simulink model "Robot"  (R2018a)
settings: Solver=VariableStepAuto  StartTime=0.0  StopTime=inf  FixedStep=1e-4  RelTol=1e-3  EnableMultiTasking=on
values from neighbouring files (symbols this model uses):
  CM730_acc_center = (4 * 9.80665)    (= 39.2266)    [CM730.m]
  CM730_acc_gain = 512 / CM730_acc_center    (= 13.0523675261)    [CM730.m]
  CM730_gyro_center = (1600 / 360 * 2 * pi)    (= 27.9252680319)    [CM730.m]
  CM730_gyro_gain = 512 / CM730_gyro_center    (= 18.3346494442)    [CM730.m]
  CM730_sample_time = 1e-3    (= 0.001)    [CM730.m]
  FSR_max = 254    [FSR.m]
  FSR_no_load = 255    [FSR.m]
  FSR_sample_time = 0.001    [FSR.m]
  FSR_scale = 1000    [FSR.m]
  g = 0    [Euler.m]
  MX106_Te = 1/1000    (= 0.001)    [MX106_init.m]
  MX28_inertia = 9e-8 * MX28_reduction^2    (= 0.0033385284)    [MX28_init.m]
  MX28_Te = 1/1000    (= 0.001)    [MX28_init.m]
  posZero_ID1 = posZero(1)    [Robot_init.m]
  posZero_ID10 = posZero(14)    [Robot_init.m]
  posZero_ID11 = posZero(9)    [Robot_init.m]
  posZero_ID12 = posZero(15)    [Robot_init.m]
  posZero_ID13 = posZero(10)    [Robot_init.m]
  posZero_ID14 = posZero(16)    [Robot_init.m]
  posZero_ID15 = posZero(11)    [Robot_init.m]
  posZero_ID16 = posZero(17)    [Robot_init.m]
  posZero_ID17 = posZero(12)    [Robot_init.m]
  posZero_ID18 = posZero(18)    [Robot_init.m]
  posZero_ID19 = posZero(19)    [Robot_init.m]
  posZero_ID2 = posZero(4)    [Robot_init.m]
  posZero_ID20 = posZero(20)    [Robot_init.m]
  posZero_ID3 = posZero(2)    [Robot_init.m]
  posZero_ID4 = posZero(5)    [Robot_init.m]
  posZero_ID5 = posZero(3)    [Robot_init.m]
  posZero_ID6 = posZero(6)    [Robot_init.m]
  posZero_ID7 = posZero(7)    [Robot_init.m]
  posZero_ID8 = posZero(13)    [Robot_init.m]
  posZero_ID9 = posZero(8)    [Robot_init.m]
  robot_chest_mass = 2385.0    (= 2385)    [Robot_init.m]
  robot_floor_friction_coeff = 0.6    [Robot_init.m]
  robot_floor_position_gain = -1e5    (= -100000)    [Robot_init.m]
  robot_floor_speed_gain = -1e3    (= -1000)    [Robot_init.m]
  robot_gravity = [0 0 0]    [Robot_init.m]
  robot_head_mass = 177.69    [Robot_init.m]
  robot_hip1_mass = 49.00    (= 49)    [Robot_init.m]
  robot_left_ankle_mass = 360.00    (= 360)    [Robot_init.m]
  robot_left_foot_mass = 267.00    (= 267)    [Robot_init.m]
  robot_left_forearm_mass = 248.00    (= 248)    [Robot_init.m]
  robot_left_hip2_mass = 358.00    (= 358)    [Robot_init.m]
  robot_left_lower_leg_mass = 129.00    (= 129)    [Robot_init.m]
  robot_left_shoulder_mass = 39.00    (= 39)    [Robot_init.m]
  robot_left_thigh_mass = 1263.00    (= 1263)    [Robot_init.m]
  robot_left_upper_arm_mass = 247.00    (= 247)    [Robot_init.m]
  robot_neck_mass = 90    [Robot_init.m]
  robot_right_ankle_mass = 360.00    (= 360)    [Robot_init.m]
  robot_right_foot_mass = 267.00    (= 267)    [Robot_init.m]
  robot_right_forearm_mass = 248.00    (= 248)    [Robot_init.m]
  robot_right_hip2_mass = 358.00    (= 358)    [Robot_init.m]
  robot_right_lower_leg_mass = 129.00    (= 129)    [Robot_init.m]
  robot_right_shoulder_mass = 39.00    (= 39)    [Robot_init.m]
  robot_right_thigh_mass = 263.00    (= 263)    [Robot_init.m]
  robot_right_upper_arm_mass = 247.00    (= 247)    [Robot_init.m]
  X = get(hObject,'Value')    [gui_kine.m]
  Y = get(hObject,'Value')    [gui_kine.m]
  Z = get(hObject,'Value')    [gui_kine.m]
libraries: sm_lib x167, fl_lib x128, nesl_utility x77, dspindex x1
(part 4 of 7)

== system Robot/Robot simulation/Left Leg/Left Foot ==
  Left Foot Axis to Back Left : sm_lib/Frames and Transforms/Rigid Transform  TranslationMethod=Cartesian  TranslationStandardOffset=0  TranslationLengthUnit=mm  TranslationStandardAxis=+Z  TranslationCartesianOffset=robot_left_foot_to_back_left_floor_tra  TranslationROffset=0  TranslationROffsetUnits=m  TranslationZOffset=0  TranslationZOffsetUnits=m  TranslationThetaOffset=0  TranslationThetaOffsetUnits=deg  RotationMethod=RotationMatrix  RotationAngleUnits=deg  RotationStandardAxis=+Z  RotationAngle=0.0  RotationArbitraryAxis=[0 0 1]  FollAlignAxisA=+X  BaseAlignAxisA=-X  FollAlignAxisB=+Z  BaseAlignAxisB=-Y  RotationSequenceAxes=FollowerAxes  RotationSequence=XYX  RotationSequenceAngles=[0 0 0]  RotationSequenceAnglesUnits=deg  RotationMatrix=robot_left_foot_to_floor_rot
  Left Foot Axis to Back Right : sm_lib/Frames and Transforms/Rigid Transform  TranslationMethod=Cartesian  TranslationStandardOffset=0  TranslationLengthUnit=mm  TranslationStandardAxis=+Z  TranslationCartesianOffset=robot_left_foot_to_back_right_floor_tra  TranslationROffset=0  TranslationROffsetUnits=m  TranslationZOffset=0  TranslationZOffsetUnits=m  TranslationThetaOffset=0  TranslationThetaOffsetUnits=deg  RotationMethod=RotationMatrix  RotationAngleUnits=deg  RotationStandardAxis=+Z  RotationAngle=0.0  RotationArbitraryAxis=[0 0 1]  FollAlignAxisA=+X  BaseAlignAxisA=-X  FollAlignAxisB=+Z  BaseAlignAxisB=-Y  RotationSequenceAxes=FollowerAxes  RotationSequence=XYX  RotationSequenceAngles=[0 0 0]  RotationSequenceAnglesUnits=deg  RotationMatrix=robot_left_foot_to_floor_rot
  Left Foot Axis to Front Left : sm_lib/Frames and Transforms/Rigid Transform  TranslationMethod=Cartesian  TranslationStandardOffset=0  TranslationLengthUnit=mm  TranslationStandardAxis=+Z  TranslationCartesianOffset=robot_left_foot_to_front_left_floor_tra  TranslationROffset=0  TranslationROffsetUnits=m  TranslationZOffset=0  TranslationZOffsetUnits=m  TranslationThetaOffset=0  TranslationThetaOffsetUnits=deg  RotationMethod=RotationMatrix  RotationAngleUnits=deg  RotationStandardAxis=+Z  RotationAngle=0.0  RotationArbitraryAxis=[0 0 1]  FollAlignAxisA=+X  BaseAlignAxisA=-X  FollAlignAxisB=+Z  BaseAlignAxisB=-Y  RotationSequenceAxes=FollowerAxes  RotationSequence=XYX  RotationSequenceAngles=[0 0 0]  RotationSequenceAnglesUnits=deg  RotationMatrix=robot_left_foot_to_floor_rot
  Left Foot Axis to Front Right : sm_lib/Frames and Transforms/Rigid Transform  TranslationMethod=Cartesian  TranslationStandardOffset=0  TranslationLengthUnit=mm  TranslationStandardAxis=+Z  TranslationCartesianOffset=robot_left_foot_to_front_right_floor_tra  TranslationROffset=0  TranslationROffsetUnits=m  TranslationZOffset=0  TranslationZOffsetUnits=m  TranslationThetaOffset=0  TranslationThetaOffsetUnits=deg  RotationMethod=RotationMatrix  RotationAngleUnits=deg  RotationStandardAxis=+Z  RotationAngle=0.0  RotationArbitraryAxis=[0 0 1]  FollAlignAxisA=+X  BaseAlignAxisA=-X  FollAlignAxisB=+Z  BaseAlignAxisB=-Y  RotationSequenceAxes=FollowerAxes  RotationSequence=XYX  RotationSequenceAngles=[0 0 0]  RotationSequenceAnglesUnits=deg  RotationMatrix=robot_left_foot_to_floor_rot
  Left Foot Endefector : sm_lib/Frames and Transforms/Rigid Transform  TranslationMethod=Cartesian  TranslationStandardOffset=0  TranslationLengthUnit=mm  TranslationStandardAxis=+Z  TranslationCartesianOffset=robot_left_foot_Endefector_tra  TranslationROffset=0  TranslationROffsetUnits=m  TranslationZOffset=0  TranslationZOffsetUnits=m  TranslationThetaOffset=0  TranslationThetaOffsetUnits=deg  RotationMethod=RotationMatrix  RotationAngleUnits=deg  RotationStandardAxis=+Z  RotationAngle=0.0  RotationArbitraryAxis=[0 0 1]  FollAlignAxisA=+X  BaseAlignAxisA=-X  FollAlignAxisB=+Z  BaseAlignAxisB=-Y  RotationSequenceAxes=FollowerAxes  RotationSequence=XYX  RotationSequenceAngles=[0 0 0]  RotationSequenceAnglesUnits=deg  RotationMatrix=robot_left_foot_Endefector_rot
  Solid : sm_lib/Body Elements/Solid  InertiaType=Custom  Mass=robot_left_foot_mass  MassUnits=g  CenterOfMass=robot_left_foot_to_center_mass  CenterOfMassUnits=mm  MomentsOfInertia=robot_left_foot_moment_inertia  MomentsOfInertiaUnits=g*mm^2  ProductsOfInertia=robot_left_foot_product_inertia  ProductsOfInertiaUnits=g*mm^2  DensityBased=on  Density=1000  DensityUnits=kg/(m^3)  DoExposeReferenceFrame=on  SerializedFrames=<Frames/>  GraphicType=FromGeometry  MarkerShape=Sphere  MarkerSize=10  MarkerSizeUnits=m  GraphicVisPropType=SimpleVisualProperties  GraphicDiffuseColor=[0.5 0.5 0.5]  GraphicSpecularColor=[0.5 0.5 0.5 1.0]  GraphicAmbientColor=[0.15 0.15 0.15 1.0]  GraphicEmissiveColor=[0.0 0.0 0.0 1.0]  GraphicShininess=75  GraphicOpacity=1.0  GeometryShape=FromFile  RectangleSize=[1 1]  RectangleSizeUnits=m  BrickDimensions=[1 1 1]  BrickDimensionUnits=m  CylinderRadius=1  CylinderRadiusUnits=m  CylinderLength=1  CylinderLengthUnits=m  SphereRadius=1  SphereRadiusUnits=m  EllipsoidRadii=[1 1 1]  EllipsoidRadiiUnits=m  ExtrusionCrossSection=[1 1; -1 1; -1 -1; 1 -1]  ExtrusionCrossSectionUnits=m  ExtrusionLength=1  ExtrusionLengthUnits=m  PolygonNumSides=3  PolygonOuterRadius=1  PolygonOuterRadiusUnits=m  ExtGeomFileType=STL  ExtGeomFileName=\STL\Left_Foot.STL  ExtGeomFileUnits=mm  RevolutionCrossSection=[1 1; 1 -1; 2 -1; 2 1]  RevolutionCrossSectionUnits=m  RevolutionExtent=Full  RevolutionAngle=180  RevolutionAngleUnits=deg
  Foot : PMIOPort  Side=Left
  Front Left : PMIOPort  Port=2  Side=Right
  Front Right : PMIOPort  Port=3  Side=Right
  Back Right : PMIOPort  Port=4  Side=Right
  Back Left : PMIOPort  Port=5  Side=Right
  EndEfector : PMIOPort  Port=6  Side=Right
  connections:
  Foot/RConn1 -- Left Foot Axis to Back Right/LConn1 -- Left Foot Axis to Front Left/LConn1 -- Left Foot Endefector/LConn1 -- Left Foot Axis to Front Right/LConn1 -- Left Foot Axis to Back Left/LConn1 -- Solid/RConn1
  Front Left/RConn1 -- Left Foot Axis to Front Left/RConn1
  Front Right/RConn1 -- Left Foot Axis to Front Right/RConn1
  Back Right/RConn1 -- Left Foot Axis to Back Right/RConn1
  Back Left/RConn1 -- Left Foot Axis to Back Left/RConn1
  EndEfector/RConn1 -- Left Foot Endefector/RConn1

== system Robot/Robot simulation/Left Leg/Left Hip Pitch (12) ==
  Inertia : sm_lib/Body Elements/Inertia  InertiaType=Custom  Mass=1  MassUnits=g  CenterOfMass=[0 0 0]  CenterOfMassUnits=m  MomentsOfInertia=[0 0 MX28_inertia]  MomentsOfInertiaUnits=kg*m^2  ProductsOfInertia=[0 0 0]  ProductsOfInertiaUnits=kg*m^2  GraphicType=Marker  MarkerShape=Inertia  MarkerSize=20  GraphicVisPropType=SimpleVisualProperties  GraphicDiffuseColor=[0.5 0.5 0.5]  GraphicSpecularColor=[0.5 0.5 0.5 1.0]  GraphicAmbientColor=[0.15 0.15 0.15 1.0]  GraphicEmissiveColor=[0.0 0.0 0.0 1.0]  GraphicShininess=75  GraphicOpacity=1.0
  MX106 Command : DataStoreRead  DataStoreName=MX106_ID12  SampleTime=MX106_Te  DataStoreElements=MX106_ID12.CW_angle_limit#MX106_ID12.CCW_angle_limit#MX106_ID12.torque_enable#MX106_ID12.D_gain#MX106_ID12.I_gain#MX106_ID12.P_gain#MX106_ID12.goal_position#MX106_ID12.moving_speed#MX106_ID12.torque_limit
  MX106 State : DataStoreWrite  DataStoreName=MX106_ID12  DataStoreElements=MX106_ID12.present_position#MX106_ID12.present_speed#MX106_ID12.present_load#MX106_ID12.moving#MX106_ID12.pwm
  Model : ModelReference  ModelNameDialog=MX106.slx  SimulationMode=Normal  ModelReferenceVersion=1.67
  Position converter : nesl_utility/PS-Simulink Converter  PhysicalDomain=network_engine_domain  SubClassName=ps_output  LeftPortType=input  RightPortType=output  PseudoPeriodic=off  Frequencies=[]  Unit=rad  AffineConversion=off
  Revolute Joint : sm_lib/Joints/Revolute Joint  SenseConstraintForce=off  SenseConstraintForceX=off  SenseConstraintForceY=off  SenseConstraintForceZ=off  SenseConstraintTorque=off  SenseConstraintTorqueX=off  SenseConstraintTorqueY=off  SenseConstraintTorqueZ=off  SenseTotalForce=off  SenseTotalForceX=off  SenseTotalForceY=off  SenseTotalForceZ=off  SenseTotalTorque=off  SenseTotalTorqueX=off  SenseTotalTorqueY=off  SenseTotalTorqueZ=off  CompositeWrenchDir=FollowerOnBase  CompositeWrenchFrame=BaseFrame  EquilibriumPosition=0  EquilibriumPositionUnits=deg  SpringStiffness=0  SpringStiffnessUnits=N*m/deg  DampingCoefficient=MX28_lub_friction  DampingCoefficientUnits=N*m/(rad/s)  TorqueActuationMode=InputTorque  MotionActuationMode=ComputedMotion  SensePosition=on  SenseVelocity=on  SenseAcceleration=off  SenseTorqueForce=off  PositionTargetSpecify=on  PositionTargetPriority=High  PositionTargetValue=MX28_init_position  PositionTargetValueUnits=rad  VelocityTargetSpecify=on  VelocityTargetPriority=High  VelocityTargetValue=MX28_init_speed  VelocityTargetValueUnits=rad/s
  Speed converter : nesl_utility/PS-Simulink Converter  PhysicalDomain=network_engine_domain  SubClassName=ps_output  LeftPortType=input  RightPortType=output  PseudoPeriodic=off  Frequencies=[]  Unit=rad/s  AffineConversion=off
  Torque converter : nesl_utility/Simulink-PS Converter  PhysicalDomain=network_engine_domain  SubClassName=ps_input  LeftPortType=input  RightPortType=output  PseudoPeriodic=off  Frequencies=[]  NoiseDistribution=none  NoiseParameters=[]  Unit=N*m  AffineConversion=off  FilteringAndDerivatives=zero  SimscapeFilterOrder=1  InputFilterTimeConstant=0.001  UdotUserProvided=1
  Base : PMIOPort  Side=Left
  Axis : PMIOPort  Port=2  Side=Right
  wires:
  Model/4 -> MX106 State/3
  Model/2 -> MX106 State/1
  Model/5 -> MX106 State/4
  Model/3 -> MX106 State/2
  MX106 Command/3 -> Model/5
  MX106 Command/6 -> Model/8
  MX106 Command/4 -> Model/6
  MX106 Command/5 -> Model/7
  MX106 Command/7 -> Model/9
  MX106 Command/2 -> Model/4
  MX106 Command/1 -> Model/3
  Speed converter/1 -> Model/1
  Position converter/1 -> Model/2
  Model/6 -> MX106 State/5
  MX106 Command/8 -> Model/10
  MX106 Command/9 -> Model/11
  Model/1 -> Torque converter/1
  connections:
  Axis/RConn1 -- Revolute Joint/RConn1 -- Inertia/RConn1
  Revolute Joint/LConn1 -- Base/RConn1
  Revolute Joint/RConn3 -- Speed converter/LConn1
  Revolute Joint/RConn2 -- Position converter/LConn1
  Revolute Joint/LConn2 -- Torque converter/RConn1

== system Robot/Robot simulation/Left Leg/Left Hip Roll ==
  Left Hip Roll Base to Left Hip Pitch Base : sm_lib/Frames and Transforms/Rigid Transform  TranslationMethod=Cartesian  TranslationStandardOffset=0  TranslationLengthUnit=mm  TranslationStandardAxis=+Z  TranslationCartesianOffset=robot_left_hip2_to_left_thigh_tra  TranslationROffset=0  TranslationROffsetUnits=m  TranslationZOffset=0  TranslationZOffsetUnits=m  TranslationThetaOffset=0  TranslationThetaOffsetUnits=deg  RotationMethod=RotationMatrix  RotationAngleUnits=deg  RotationStandardAxis=+Z  RotationAngle=0  RotationArbitraryAxis=[0 0 1]  FollAlignAxisA=+Y  BaseAlignAxisA=+Y  FollAlignAxisB=+X  BaseAlignAxisB=+Z  RotationSequenceAxes=FollowerAxes  RotationSequence=XYX  RotationSequenceAngles=[0 0 0]  RotationSequenceAnglesUnits=deg  RotationMatrix=robot_left_hip2_to_left_thigh_rot
  Solid : sm_lib/Body Elements/Solid  InertiaType=Custom  Mass=robot_left_hip2_mass  MassUnits=g  CenterOfMass=robot_left_hip2_to_center_mass  CenterOfMassUnits=mm  MomentsOfInertia=robot_left_hip2_moment_inertia  MomentsOfInertiaUnits=g*mm^2  ProductsOfInertia=robot_left_hip2_product_inertia  ProductsOfInertiaUnits=g*mm^2  DensityBased=on  Density=1000  DensityUnits=kg/(m^3)  DoExposeReferenceFrame=on  SerializedFrames=<Frames/>  GraphicType=FromGeometry  MarkerShape=Sphere  MarkerSize=10  MarkerSizeUnits=m  GraphicVisPropType=SimpleVisualProperties  GraphicDiffuseColor=[0.5 0.5 0.5]  GraphicSpecularColor=[0.5 0.5 0.5 1.0]  GraphicAmbientColor=[0.15 0.15 0.15 1.0]  GraphicEmissiveColor=[0.0 0.0 0.0 1.0]  GraphicShininess=75  GraphicOpacity=1.0  GeometryShape=FromFile  RectangleSize=[1 1]  RectangleSizeUnits=m  BrickDimensions=[1 1 1]  BrickDimensionUnits=mm  CylinderRadius=1  CylinderRadiusUnits=m  CylinderLength=1  CylinderLengthUnits=m  SphereRadius=1  SphereRadiusUnits=m  EllipsoidRadii=[1 1 1]  EllipsoidRadiiUnits=m  ExtrusionCrossSection=[1 1; -1 1; -1 -1; 1 -1]  ExtrusionCrossSectionUnits=m  ExtrusionLength=1  ExtrusionLengthUnits=m  PolygonNumSides=3  PolygonOuterRadius=1  PolygonOuterRadiusUnits=m  ExtGeomFileType=STL  ExtGeomFileName=\STL\Left_Hip2.STL  ExtGeomFileUnits=mm  RevolutionCrossSection=[1 1; 1 -1; 2 -1; 2 1]  RevolutionCrossSectionUnits=m  RevolutionExtent=Full  RevolutionAngle=180  RevolutionAngleUnits=deg
  Left Hip Roll : PMIOPort  Side=Left
  Left Hip Pitch : PMIOPort  Port=2  Side=Right
  connections:
  Left Hip Roll Base to Left Hip Pitch Base/LConn1 -- Solid/RConn1 -- Left Hip Roll/RConn1
  Left Hip Roll Base to Left Hip Pitch Base/RConn1 -- Left Hip Pitch/RConn1

== system Robot/Robot simulation/Left Leg/Left Hip Roll (10) ==
  Inertia : sm_lib/Body Elements/Inertia  InertiaType=Custom  Mass=1  MassUnits=g  CenterOfMass=[0 0 0]  CenterOfMassUnits=m  MomentsOfInertia=[0 0 MX28_inertia]  MomentsOfInertiaUnits=kg*m^2  ProductsOfInertia=[0 0 0]  ProductsOfInertiaUnits=kg*m^2  GraphicType=Marker  MarkerShape=Inertia  MarkerSize=20  GraphicVisPropType=SimpleVisualProperties  GraphicDiffuseColor=[0.5 0.5 0.5]  GraphicSpecularColor=[0.5 0.5 0.5 1.0]  GraphicAmbientColor=[0.15 0.15 0.15 1.0]  GraphicEmissiveColor=[0.0 0.0 0.0 1.0]  GraphicShininess=75  GraphicOpacity=1.0
  MX106 Command : DataStoreRead  DataStoreName=MX106_ID10  SampleTime=MX106_Te  DataStoreElements=MX106_ID10.CW_angle_limit#MX106_ID10.CCW_angle_limit#MX106_ID10.torque_enable#MX106_ID10.D_gain#MX106_ID10.I_gain#MX106_ID10.P_gain#MX106_ID10.goal_position#MX106_ID10.moving_speed#MX106_ID10.torque_limit
  MX106 State : DataStoreWrite  DataStoreName=MX106_ID10  DataStoreElements=MX106_ID10.present_position#MX106_ID10.present_speed#MX106_ID10.present_load#MX106_ID10.moving#MX106_ID10.pwm
  Model : ModelReference  ModelNameDialog=MX106.slx  SimulationMode=Normal  ModelReferenceVersion=1.67
  Position converter : nesl_utility/PS-Simulink Converter  PhysicalDomain=network_engine_domain  SubClassName=ps_output  LeftPortType=input  RightPortType=output  PseudoPeriodic=off  Frequencies=[]  Unit=rad  AffineConversion=off
  Revolute Joint : sm_lib/Joints/Revolute Joint  SenseConstraintForce=off  SenseConstraintForceX=off  SenseConstraintForceY=off  SenseConstraintForceZ=off  SenseConstraintTorque=off  SenseConstraintTorqueX=off  SenseConstraintTorqueY=off  SenseConstraintTorqueZ=off  SenseTotalForce=off  SenseTotalForceX=off  SenseTotalForceY=off  SenseTotalForceZ=off  SenseTotalTorque=off  SenseTotalTorqueX=off  SenseTotalTorqueY=off  SenseTotalTorqueZ=off  CompositeWrenchDir=FollowerOnBase  CompositeWrenchFrame=BaseFrame  EquilibriumPosition=0  EquilibriumPositionUnits=deg  SpringStiffness=0  SpringStiffnessUnits=N*m/deg  DampingCoefficient=MX28_lub_friction  DampingCoefficientUnits=N*m/(rad/s)  TorqueActuationMode=InputTorque  MotionActuationMode=ComputedMotion  SensePosition=on  SenseVelocity=on  SenseAcceleration=off  SenseTorqueForce=off  PositionTargetSpecify=on  PositionTargetPriority=High  PositionTargetValue=MX28_init_position  PositionTargetValueUnits=rad  VelocityTargetSpecify=on  VelocityTargetPriority=High  VelocityTargetValue=MX28_init_speed  VelocityTargetValueUnits=rad/s
  Speed converter : nesl_utility/PS-Simulink Converter  PhysicalDomain=network_engine_domain  SubClassName=ps_output  LeftPortType=input  RightPortType=output  PseudoPeriodic=off  Frequencies=[]  Unit=rad/s  AffineConversion=off
  Torque converter : nesl_utility/Simulink-PS Converter  PhysicalDomain=network_engine_domain  SubClassName=ps_input  LeftPortType=input  RightPortType=output  PseudoPeriodic=off  Frequencies=[]  NoiseDistribution=none  NoiseParameters=[]  Unit=N*m  AffineConversion=off  FilteringAndDerivatives=zero  SimscapeFilterOrder=1  InputFilterTimeConstant=0.001  UdotUserProvided=1
  Base : PMIOPort  Side=Left
  Axis : PMIOPort  Port=2  Side=Right
  wires:
  Model/4 -> MX106 State/3
  Model/2 -> MX106 State/1
  Model/5 -> MX106 State/4
  Model/3 -> MX106 State/2
  MX106 Command/3 -> Model/5
  MX106 Command/6 -> Model/8
  MX106 Command/4 -> Model/6
  MX106 Command/5 -> Model/7
  MX106 Command/7 -> Model/9
  MX106 Command/2 -> Model/4
  MX106 Command/1 -> Model/3
  Position converter/1 -> Model/2
  Speed converter/1 -> Model/1
  Model/6 -> MX106 State/5
  MX106 Command/8 -> Model/10
  MX106 Command/9 -> Model/11
  Model/1 -> Torque converter/1
  connections:
  Axis/RConn1 -- Revolute Joint/RConn1 -- Inertia/RConn1
  Revolute Joint/LConn1 -- Base/RConn1
  Revolute Joint/RConn3 -- Speed converter/LConn1
  Revolute Joint/RConn2 -- Position converter/LConn1
  Revolute Joint/LConn2 -- Torque converter/RConn1

== system Robot/Robot simulation/Left Leg/Left Hip Yaw ==
  Left Hip Yaw Axis to Left Hip Roll Axis : sm_lib/Frames and Transforms/Rigid Transform  TranslationMethod=Cartesian  TranslationStandardOffset=0  TranslationLengthUnit=mm  TranslationStandardAxis=+Z  TranslationCartesianOffset=robot_hip1_to_hip2_tra  TranslationROffset=0  TranslationROffsetUnits=m  TranslationZOffset=0  TranslationZOffsetUnits=m  TranslationThetaOffset=0  TranslationThetaOffsetUnits=deg  RotationMethod=RotationMatrix  RotationAngleUnits=deg  RotationStandardAxis=+Z  RotationAngle=0  RotationArbitraryAxis=[0 0 1]  FollAlignAxisA=+Y  BaseAlignAxisA=+Z  FollAlignAxisB=+X  BaseAlignAxisB=-Y  RotationSequenceAxes=FollowerAxes  RotationSequence=XYX  RotationSequenceAngles=[0 0 0]  RotationSequenceAnglesUnits=deg  RotationMatrix=robot_hip1_to_hip2_rot
  Solid : sm_lib/Body Elements/Solid  InertiaType=Custom  Mass=robot_hip1_mass  MassUnits=g  CenterOfMass=robot_hip1_to_center_mass  CenterOfMassUnits=mm  MomentsOfInertia=robot_hip1_moment_inertia  MomentsOfInertiaUnits=g*mm^2  ProductsOfInertia=robot_hip1_product_inertia  ProductsOfInertiaUnits=g*mm^2  DensityBased=on  Density=1000  DensityUnits=kg/(m^3)  DoExposeReferenceFrame=on  SerializedFrames=<Frames/>  GraphicType=FromGeometry  MarkerShape=Sphere  MarkerSize=10  MarkerSizeUnits=m  GraphicVisPropType=SimpleVisualProperties  GraphicDiffuseColor=[0.5 0.5 0.5]  GraphicSpecularColor=[0.5 0.5 0.5 1.0]  GraphicAmbientColor=[0.15 0.15 0.15 1.0]  GraphicEmissiveColor=[0.0 0.0 0.0 1.0]  GraphicShininess=75  GraphicOpacity=1.0  GeometryShape=FromFile  RectangleSize=[1 1]  RectangleSizeUnits=m  BrickDimensions=[1 1 1]  BrickDimensionUnits=mm  CylinderRadius=1  CylinderRadiusUnits=m  CylinderLength=1  CylinderLengthUnits=m  SphereRadius=1  SphereRadiusUnits=m  EllipsoidRadii=[1 1 1]  EllipsoidRadiiUnits=m  ExtrusionCrossSection=[1 1; -1 1; -1 -1; 1 -1]  ExtrusionCrossSectionUnits=m  ExtrusionLength=1  ExtrusionLengthUnits=m  PolygonNumSides=3  PolygonOuterRadius=1  PolygonOuterRadiusUnits=m  ExtGeomFileType=STL  ExtGeomFileName=\STL\Hip1.STL  ExtGeomFileUnits=mm  RevolutionCrossSection=[1 1; 1 -1; 2 -1; 2 1]  RevolutionCrossSectionUnits=m  RevolutionExtent=Full  RevolutionAngle=180  RevolutionAngleUnits=deg
  Left Hip Yaw : PMIOPort  Side=Left
  Left Hip Roll : PMIOPort  Port=2  Side=Right
  connections:
  Left Hip Yaw/RConn1 -- Solid/RConn1 -- Left Hip Yaw Axis to Left Hip Roll Axis/LConn1
  Left Hip Yaw Axis to Left Hip Roll Axis/RConn1 -- Left Hip Roll/RConn1

== system Robot/Robot simulation/Left Leg/Left Hip Yaw (8) ==
  Inertia : sm_lib/Body Elements/Inertia  InertiaType=Custom  Mass=1  MassUnits=g  CenterOfMass=[0 0 0]  CenterOfMassUnits=m  MomentsOfInertia=[0 0 MX28_inertia]  MomentsOfInertiaUnits=kg*m^2  ProductsOfInertia=[0 0 0]  ProductsOfInertiaUnits=kg*m^2  GraphicType=Marker  MarkerShape=Inertia  MarkerSize=20  GraphicVisPropType=SimpleVisualProperties  GraphicDiffuseColor=[0.5 0.5 0.5]  GraphicSpecularColor=[0.5 0.5 0.5 1.0]  GraphicAmbientColor=[0.15 0.15 0.15 1.0]  GraphicEmissiveColor=[0.0 0.0 0.0 1.0]  GraphicShininess=75  GraphicOpacity=1.0
  MX106 Command : DataStoreRead  DataStoreName=MX106_ID8  SampleTime=MX106_Te  DataStoreElements=MX106_ID8.CW_angle_limit#MX106_ID8.CCW_angle_limit#MX106_ID8.torque_enable#MX106_ID8.D_gain#MX106_ID8.I_gain#MX106_ID8.P_gain#MX106_ID8.goal_position#MX106_ID8.moving_speed#MX106_ID8.torque_limit
  MX106 State : DataStoreWrite  DataStoreName=MX106_ID8  DataStoreElements=MX106_ID8.present_position#MX106_ID8.present_speed#MX106_ID8.present_load#MX106_ID8.moving#MX106_ID8.pwm
  Model : ModelReference  ModelNameDialog=MX106.slx  SimulationMode=Normal  ModelReferenceVersion=1.67
  Position converter : nesl_utility/PS-Simulink Converter  PhysicalDomain=network_engine_domain  SubClassName=ps_output  LeftPortType=input  RightPortType=output  PseudoPeriodic=off  Frequencies=[]  Unit=rad  AffineConversion=off
  Revolute Joint : sm_lib/Joints/Revolute Joint  SenseConstraintForce=off  SenseConstraintForceX=off  SenseConstraintForceY=off  SenseConstraintForceZ=off  SenseConstraintTorque=off  SenseConstraintTorqueX=off  SenseConstraintTorqueY=off  SenseConstraintTorqueZ=off  SenseTotalForce=off  SenseTotalForceX=off  SenseTotalForceY=off  SenseTotalForceZ=off  SenseTotalTorque=off  SenseTotalTorqueX=off  SenseTotalTorqueY=off  SenseTotalTorqueZ=off  CompositeWrenchDir=FollowerOnBase  CompositeWrenchFrame=BaseFrame  EquilibriumPosition=0  EquilibriumPositionUnits=deg  SpringStiffness=0  SpringStiffnessUnits=N*m/deg  DampingCoefficient=MX28_lub_friction  DampingCoefficientUnits=N*m/(rad/s)  TorqueActuationMode=InputTorque  MotionActuationMode=ComputedMotion  SensePosition=on  SenseVelocity=on  SenseAcceleration=off  SenseTorqueForce=off  PositionTargetSpecify=on  PositionTargetPriority=High  PositionTargetValue=MX28_init_position  PositionTargetValueUnits=rad  VelocityTargetSpecify=on  VelocityTargetPriority=High  VelocityTargetValue=MX28_init_speed  VelocityTargetValueUnits=rad/s
  Speed converter : nesl_utility/PS-Simulink Converter  PhysicalDomain=network_engine_domain  SubClassName=ps_output  LeftPortType=input  RightPortType=output  PseudoPeriodic=off  Frequencies=[]  Unit=rad/s  AffineConversion=off
  Torque converter : nesl_utility/Simulink-PS Converter  PhysicalDomain=network_engine_domain  SubClassName=ps_input  LeftPortType=input  RightPortType=output  PseudoPeriodic=off  Frequencies=[]  NoiseDistribution=none  NoiseParameters=[]  Unit=N*m  AffineConversion=off  FilteringAndDerivatives=zero  SimscapeFilterOrder=1  InputFilterTimeConstant=0.001  UdotUserProvided=1
  Base : PMIOPort  Side=Left
  Axis : PMIOPort  Port=2  Side=Right
  wires:
  Model/4 -> MX106 State/3
  Model/2 -> MX106 State/1
  Model/5 -> MX106 State/4
  Model/3 -> MX106 State/2
  MX106 Command/3 -> Model/5
  MX106 Command/6 -> Model/8
  MX106 Command/4 -> Model/6
  MX106 Command/5 -> Model/7
  MX106 Command/7 -> Model/9
  MX106 Command/2 -> Model/4
  MX106 Command/1 -> Model/3
  Speed converter/1 -> Model/1
  Position converter/1 -> Model/2
  Model/6 -> MX106 State/5
  MX106 Command/8 -> Model/10
  MX106 Command/9 -> Model/11
  Model/1 -> Torque converter/1
  connections:
  Axis/RConn1 -- Revolute Joint/RConn1 -- Inertia/RConn1
  Revolute Joint/LConn1 -- Base/RConn1
  Revolute Joint/RConn3 -- Speed converter/LConn1
  Revolute Joint/RConn2 -- Position converter/LConn1
  Revolute Joint/LConn2 -- Torque converter/RConn1

== system Robot/Robot simulation/Left Leg/Left Knee (14) ==
  Inertia : sm_lib/Body Elements/Inertia  InertiaType=Custom  Mass=1  MassUnits=g  CenterOfMass=[0 0 0]  CenterOfMassUnits=m  MomentsOfInertia=[0 0 MX28_inertia]  MomentsOfInertiaUnits=kg*m^2  ProductsOfInertia=[0 0 0]  ProductsOfInertiaUnits=kg*m^2  GraphicType=Marker  MarkerShape=Inertia  MarkerSize=20  GraphicVisPropType=SimpleVisualProperties  GraphicDiffuseColor=[0.5 0.5 0.5]  GraphicSpecularColor=[0.5 0.5 0.5 1.0]  GraphicAmbientColor=[0.15 0.15 0.15 1.0]  GraphicEmissiveColor=[0.0 0.0 0.0 1.0]  GraphicShininess=75  GraphicOpacity=1.0
  MX106 Command : DataStoreRead  DataStoreName=MX106_ID14  SampleTime=MX106_Te  DataStoreElements=MX106_ID14.CW_angle_limit#MX106_ID14.CCW_angle_limit#MX106_ID14.torque_enable#MX106_ID14.D_gain#MX106_ID14.I_gain#MX106_ID14.P_gain#MX106_ID14.goal_position#MX106_ID14.moving_speed#MX106_ID14.torque_limit
  MX106 State : DataStoreWrite  DataStoreName=MX106_ID14  DataStoreElements=MX106_ID14.present_position#MX106_ID14.present_speed#MX106_ID14.present_load#MX106_ID14.moving#MX106_ID14.pwm
  Model : ModelReference  ModelNameDialog=MX106.slx  SimulationMode=Normal  ModelReferenceVersion=1.67
  Position converter : nesl_utility/PS-Simulink Converter  PhysicalDomain=network_engine_domain  SubClassName=ps_output  LeftPortType=input  RightPortType=output  PseudoPeriodic=off  Frequencies=[]  Unit=rad  AffineConversion=off
  Revolute Joint : sm_lib/Joints/Revolute Joint  SenseConstraintForce=off  SenseConstraintForceX=off  SenseConstraintForceY=off  SenseConstraintForceZ=off  SenseConstraintTorque=off  SenseConstraintTorqueX=off  SenseConstraintTorqueY=off  SenseConstraintTorqueZ=off  SenseTotalForce=off  SenseTotalForceX=off  SenseTotalForceY=off  SenseTotalForceZ=off  SenseTotalTorque=off  SenseTotalTorqueX=off  SenseTotalTorqueY=off  SenseTotalTorqueZ=off  CompositeWrenchDir=FollowerOnBase  CompositeWrenchFrame=BaseFrame  EquilibriumPosition=0  EquilibriumPositionUnits=deg  SpringStiffness=0  SpringStiffnessUnits=N*m/deg  DampingCoefficient=MX28_lub_friction  DampingCoefficientUnits=N*m/(rad/s)  TorqueActuationMode=InputTorque  MotionActuationMode=ComputedMotion  SensePosition=on  SenseVelocity=on  SenseAcceleration=off  SenseTorqueForce=off  PositionTargetSpecify=on  PositionTargetPriority=High  PositionTargetValue=MX28_init_position  PositionTargetValueUnits=rad  VelocityTargetSpecify=on  VelocityTargetPriority=High  VelocityTargetValue=MX28_init_speed  VelocityTargetValueUnits=rad/s
  Speed converter : nesl_utility/PS-Simulink Converter  PhysicalDomain=network_engine_domain  SubClassName=ps_output  LeftPortType=input  RightPortType=output  PseudoPeriodic=off  Frequencies=[]  Unit=rad/s  AffineConversion=off
  Torque converter : nesl_utility/Simulink-PS Converter  PhysicalDomain=network_engine_domain  SubClassName=ps_input  LeftPortType=input  RightPortType=output  PseudoPeriodic=off  Frequencies=[]  NoiseDistribution=none  NoiseParameters=[]  Unit=N*m  AffineConversion=off  FilteringAndDerivatives=zero  SimscapeFilterOrder=1  InputFilterTimeConstant=0.001  UdotUserProvided=1
  Base : PMIOPort  Side=Left
  Axis : PMIOPort  Port=2  Side=Right
  wires:
  Model/4 -> MX106 State/3
  Model/2 -> MX106 State/1
  Model/5 -> MX106 State/4
  Model/3 -> MX106 State/2
  MX106 Command/3 -> Model/5
  MX106 Command/6 -> Model/8
  MX106 Command/4 -> Model/6
  MX106 Command/5 -> Model/7
  MX106 Command/7 -> Model/9
  MX106 Command/2 -> Model/4
  MX106 Command/1 -> Model/3
  Speed converter/1 -> Model/1
  Position converter/1 -> Model/2
  Model/6 -> MX106 State/5
  MX106 Command/8 -> Model/10
  MX106 Command/9 -> Model/11
  Model/1 -> Torque converter/1
  connections:
  Axis/RConn1 -- Revolute Joint/RConn1 -- Inertia/RConn1
  Revolute Joint/LConn1 -- Base/RConn1
  Revolute Joint/RConn3 -- Speed converter/LConn1
  Revolute Joint/RConn2 -- Position converter/LConn1
  Revolute Joint/LConn2 -- Torque converter/RConn1

== system Robot/Robot simulation/Left Leg/Left Lower Leg ==
  Left Lower Leg Axis to Left Ankle  Axis : sm_lib/Frames and Transforms/Rigid Transform  TranslationMethod=Cartesian  TranslationStandardOffset=0  TranslationLengthUnit=mm  TranslationStandardAxis=+Z  TranslationCartesianOffset=robot_left_lower_leg_to_left_ankle_tra  TranslationROffset=0  TranslationROffsetUnits=m  TranslationZOffset=0  TranslationZOffsetUnits=m  TranslationThetaOffset=0  TranslationThetaOffsetUnits=deg  RotationMethod=RotationMatrix  RotationAngleUnits=deg  RotationStandardAxis=+Z  RotationAngle=0  RotationArbitraryAxis=[0 0 1]  FollAlignAxisA=+X  BaseAlignAxisA=+Y  FollAlignAxisB=+Y  BaseAlignAxisB=+Z  RotationSequenceAxes=FollowerAxes  RotationSequence=XYX  RotationSequenceAngles=[0 0 0]  RotationSequenceAnglesUnits=deg  RotationMatrix=robot_left_lower_leg_to_left_ankle_rot
  Solid : sm_lib/Body Elements/Solid  InertiaType=Custom  Mass=robot_left_lower_leg_mass  MassUnits=g  CenterOfMass=robot_left_lower_leg_to_center_mass  CenterOfMassUnits=mm  MomentsOfInertia=robot_left_lower_leg_moment_inertia  MomentsOfInertiaUnits=g*mm^2  ProductsOfInertia=robot_left_lower_leg_product_inertia  ProductsOfInertiaUnits=g*mm^2  DensityBased=on  Density=1000  DensityUnits=kg/(m^3)  DoExposeReferenceFrame=on  SerializedFrames=<Frames/>  GraphicType=FromGeometry  MarkerShape=Sphere  MarkerSize=10  MarkerSizeUnits=m  GraphicVisPropType=SimpleVisualProperties  GraphicDiffuseColor=[0.5 0.5 0.5]  GraphicSpecularColor=[0.5 0.5 0.5 1.0]  GraphicAmbientColor=[0.15 0.15 0.15 1.0]  GraphicEmissiveColor=[0.0 0.0 0.0 1.0]  GraphicShininess=75  GraphicOpacity=1.0  GeometryShape=FromFile  RectangleSize=[1 1]  RectangleSizeUnits=m  BrickDimensions=[1 1 1]  BrickDimensionUnits=m  CylinderRadius=1  CylinderRadiusUnits=m  CylinderLength=1  CylinderLengthUnits=m  SphereRadius=1  SphereRadiusUnits=m  EllipsoidRadii=[1 1 1]  EllipsoidRadiiUnits=m  ExtrusionCrossSection=[1 1; -1 1; -1 -1; 1 -1]  ExtrusionCrossSectionUnits=m  ExtrusionLength=1  ExtrusionLengthUnits=m  PolygonNumSides=3  PolygonOuterRadius=1  PolygonOuterRadiusUnits=m  ExtGeomFileType=STL  ExtGeomFileName=\STL\Left_Lower_Leg.STL  ExtGeomFileUnits=mm  RevolutionCrossSection=[1 1; 1 -1; 2 -1; 2 1]  RevolutionCrossSectionUnits=m  RevolutionExtent=Full  RevolutionAngle=180  RevolutionAngleUnits=deg
  Left Knee : PMIOPort  Side=Left
  Left Ankle Pitch : PMIOPort  Port=2  Side=Right
  connections:
  Solid/RConn1 -- Left Lower Leg Axis to Left Ankle  Axis/LConn1 -- Left Knee/RConn1
  Left Ankle Pitch/RConn1 -- Left Lower Leg Axis to Left Ankle  Axis/RConn1

== system Robot/Robot simulation/Left Leg/Left Thigh ==
  Left Hip Pitch Axis to Left Lower Leg Base : sm_lib/Frames and Transforms/Rigid Transform  TranslationMethod=Cartesian  TranslationStandardOffset=0  TranslationLengthUnit=mm  TranslationStandardAxis=+Z  TranslationCartesianOffset=robot_left_thigh_to_left_lower_leg_tra  TranslationROffset=0  TranslationROffsetUnits=m  TranslationZOffset=0  TranslationZOffsetUnits=m  TranslationThetaOffset=0  TranslationThetaOffsetUnits=deg  RotationMethod=RotationMatrix  RotationAngleUnits=deg  RotationStandardAxis=+Z  RotationAngle=0  RotationArbitraryAxis=[0 0 1]  FollAlignAxisA=+X  BaseAlignAxisA=+Y  FollAlignAxisB=+Y  BaseAlignAxisB=+Z  RotationSequenceAxes=FollowerAxes  RotationSequence=XYX  RotationSequenceAngles=[0 0 0]  RotationSequenceAnglesUnits=deg  RotationMatrix=robot_left_thigh_to_left_lower_leg_rot
  Solid : sm_lib/Body Elements/Solid  InertiaType=Custom  Mass=robot_left_thigh_mass  MassUnits=g  CenterOfMass=robot_left_thigh_to_center_mass  CenterOfMassUnits=mm  MomentsOfInertia=robot_left_thigh_moment_inertia  MomentsOfInertiaUnits=g*mm^2  ProductsOfInertia=robot_left_thigh_product_inertia  ProductsOfInertiaUnits=g*mm^2  DensityBased=on  Density=1000  DensityUnits=kg/(m^3)  DoExposeReferenceFrame=on  SerializedFrames=<Frames/>  GraphicType=FromGeometry  MarkerShape=Sphere  MarkerSize=10  MarkerSizeUnits=m  GraphicVisPropType=SimpleVisualProperties  GraphicDiffuseColor=[0.5 0.5 0.5]  GraphicSpecularColor=[0.5 0.5 0.5 1.0]  GraphicAmbientColor=[0.15 0.15 0.15 1.0]  GraphicEmissiveColor=[0.0 0.0 0.0 1.0]  GraphicShininess=75  GraphicOpacity=1.0  GeometryShape=FromFile  RectangleSize=[1 1]  RectangleSizeUnits=m  BrickDimensions=[1 1 1]  BrickDimensionUnits=m  CylinderRadius=1  CylinderRadiusUnits=m  CylinderLength=1  CylinderLengthUnits=m  SphereRadius=1  SphereRadiusUnits=m  EllipsoidRadii=[1 1 1]  EllipsoidRadiiUnits=m  ExtrusionCrossSection=[1 1; -1 1; -1 -1; 1 -1]  ExtrusionCrossSectionUnits=m  ExtrusionLength=1  ExtrusionLengthUnits=m  PolygonNumSides=3  PolygonOuterRadius=1  PolygonOuterRadiusUnits=m  ExtGeomFileType=STL  ExtGeomFileName=\STL\Left_Thigh.STL  ExtGeomFileUnits=mm  RevolutionCrossSection=[1 1; 1 -1; 2 -1; 2 1]  RevolutionCrossSectionUnits=m  RevolutionExtent=Full  RevolutionAngle=180  RevolutionAngleUnits=deg
  Left Hip Pitch : PMIOPort  Side=Left
  Left Knee : PMIOPort  Port=2  Side=Right
  connections:
  Solid/RConn1 -- Left Hip Pitch Axis to Left Lower Leg Base/LConn1 -- Left Hip Pitch/RConn1
  Left Knee/RConn1 -- Left Hip Pitch Axis to Left Lower Leg Base/RConn1

== system Robot/Robot simulation/Right Arm/Right Elbow (5) ==
  Inertia : sm_lib/Body Elements/Inertia  InertiaType=Custom  Mass=1  MassUnits=g  CenterOfMass=[0 0 0]  CenterOfMassUnits=m  MomentsOfInertia=[0 0 MX28_inertia]  MomentsOfInertiaUnits=kg*m^2  ProductsOfInertia=[0 0 0]  ProductsOfInertiaUnits=kg*m^2  GraphicType=Marker  MarkerShape=Inertia  MarkerSize=20  GraphicVisPropType=SimpleVisualProperties  GraphicDiffuseColor=[0.5 0.5 0.5]  GraphicSpecularColor=[0.5 0.5 0.5 1.0]  GraphicAmbientColor=[0.15 0.15 0.15 1.0]  GraphicEmissiveColor=[0.0 0.0 0.0 1.0]  GraphicShininess=75  GraphicOpacity=1.0
  MX28 Command : DataStoreRead  DataStoreName=MX28_ID5  SampleTime=MX28_Te  DataStoreElements=MX28_ID5.CW_angle_limit#MX28_ID5.CCW_angle_limit#MX28_ID5.torque_enable#MX28_ID5.D_gain#MX28_ID5.I_gain#MX28_ID5.P_gain#MX28_ID5.goal_position#MX28_ID5.moving_speed#MX28_ID5.torque_limit
  MX28 State : DataStoreWrite  DataStoreName=MX28_ID5  DataStoreElements=MX28_ID5.present_position#MX28_ID5.present_speed#MX28_ID5.present_load#MX28_ID5.moving#MX28_ID5.pwm
  Model : ModelReference  ModelNameDialog=MX28.slx  SimulationMode=Normal  ModelReferenceVersion=1.66
  Position converter : nesl_utility/PS-Simulink Converter  PhysicalDomain=network_engine_domain  SubClassName=ps_output  LeftPortType=input  RightPortType=output  PseudoPeriodic=off  Frequencies=[]  Unit=rad  AffineConversion=off
  Revolute Joint : sm_lib/Joints/Revolute Joint  SenseConstraintForce=off  SenseConstraintForceX=off  SenseConstraintForceY=off  SenseConstraintForceZ=off  SenseConstraintTorque=off  SenseConstraintTorqueX=off  SenseConstraintTorqueY=off  SenseConstraintTorqueZ=off  SenseTotalForce=off  SenseTotalForceX=off  SenseTotalForceY=off  SenseTotalForceZ=off  SenseTotalTorque=off  SenseTotalTorqueX=off  SenseTotalTorqueY=off  SenseTotalTorqueZ=off  CompositeWrenchDir=FollowerOnBase  CompositeWrenchFrame=BaseFrame  EquilibriumPosition=0  EquilibriumPositionUnits=deg  SpringStiffness=0  SpringStiffnessUnits=N*m/deg  DampingCoefficient=MX28_lub_friction  DampingCoefficientUnits=N*m/(rad/s)  TorqueActuationMode=InputTorque  MotionActuationMode=ComputedMotion  SensePosition=on  SenseVelocity=on  SenseAcceleration=off  SenseTorqueForce=off  PositionTargetSpecify=on  PositionTargetPriority=High  PositionTargetValue=MX28_init_position  PositionTargetValueUnits=rad  VelocityTargetSpecify=on  VelocityTargetPriority=High  VelocityTargetValue=MX28_init_speed  VelocityTargetValueUnits=rad/s
  Speed converter : nesl_utility/PS-Simulink Converter  PhysicalDomain=network_engine_domain  SubClassName=ps_output  LeftPortType=input  RightPortType=output  PseudoPeriodic=off  Frequencies=[]  Unit=rad/s  AffineConversion=off
  Torque converter : nesl_utility/Simulink-PS Converter  PhysicalDomain=network_engine_domain  SubClassName=ps_input  LeftPortType=input  RightPortType=output  PseudoPeriodic=off  Frequencies=[]  NoiseDistribution=none  NoiseParameters=[]  Unit=N*m  AffineConversion=off  FilteringAndDerivatives=zero  SimscapeFilterOrder=1  InputFilterTimeConstant=0.001  UdotUserProvided=1
  Base : PMIOPort  Side=Left
  Axis : PMIOPort  Port=2  Side=Right
  wires:
  Model/4 -> MX28 State/3
  Model/2 -> MX28 State/1
  Model/5 -> MX28 State/4
  Model/3 -> MX28 State/2
  MX28 Command/3 -> Model/5
  MX28 Command/6 -> Model/8
  MX28 Command/4 -> Model/6
  MX28 Command/5 -> Model/7
  MX28 Command/7 -> Model/9
  MX28 Command/2 -> Model/4
  MX28 Command/1 -> Model/3
  Speed converter/1 -> Model/1
  Position converter/1 -> Model/2
  Model/1 -> Torque converter/1
  Model/6 -> MX28 State/5
  MX28 Command/8 -> Model/10
  MX28 Command/9 -> Model/11
  connections:
  Axis/RConn1 -- Revolute Joint/RConn1 -- Inertia/RConn1
  Revolute Joint/RConn3 -- Speed converter/LConn1
  Revolute Joint/RConn2 -- Position converter/LConn1
  Revolute Joint/LConn2 -- Torque converter/RConn1
  Revolute Joint/LConn1 -- Base/RConn1

== system Robot/Robot simulation/Right Arm/Right Forearm ==
  Right Arm Endefector : sm_lib/Frames and Transforms/Rigid Transform  TranslationMethod=Cartesian  TranslationStandardOffset=0  TranslationLengthUnit=mm  TranslationStandardAxis=+Z  TranslationCartesianOffset=robot_right_arm_Endefector_tra  TranslationROffset=0  TranslationROffsetUnits=m  TranslationZOffset=0  TranslationZOffsetUnits=m  TranslationThetaOffset=0  TranslationThetaOffsetUnits=deg  RotationMethod=RotationMatrix  RotationAngleUnits=deg  RotationStandardAxis=+Z  RotationAngle=0.0  RotationArbitraryAxis=[0 0 1]  FollAlignAxisA=+X  BaseAlignAxisA=-X  FollAlignAxisB=+Z  BaseAlignAxisB=-Y  RotationSequenceAxes=FollowerAxes  RotationSequence=XYX  RotationSequenceAngles=[0 0 0]  RotationSequenceAnglesUnits=deg  RotationMatrix=robot_right_arm_Endefector_rot
  Solid : sm_lib/Body Elements/Solid  InertiaType=Custom  Mass=robot_right_forearm_mass  MassUnits=g  CenterOfMass=robot_right_forearm_to_center_mass  CenterOfMassUnits=mm  MomentsOfInertia=robot_right_forearm_moment_inertia  MomentsOfInertiaUnits=g*mm^2  ProductsOfInertia=robot_right_forearm_product_inertia  ProductsOfInertiaUnits=g*mm^2  DensityBased=on  Density=1000  DensityUnits=kg/(m^3)  DoExposeReferenceFrame=on  SerializedFrames=<Frames/>  GraphicType=FromGeometry  MarkerShape=Sphere  MarkerSize=10  MarkerSizeUnits=m  GraphicVisPropType=SimpleVisualProperties  GraphicDiffuseColor=[0.5 0.5 0.5]  GraphicSpecularColor=[0.5 0.5 0.5 1.0]  GraphicAmbientColor=[0.15 0.15 0.15 1.0]  GraphicEmissiveColor=[0.0 0.0 0.0 1.0]  GraphicShininess=75  GraphicOpacity=1.0  GeometryShape=FromFile  RectangleSize=[1 1]  RectangleSizeUnits=m  BrickDimensions=[1 1 1]  BrickDimensionUnits=m  CylinderRadius=1  CylinderRadiusUnits=m  CylinderLength=1  CylinderLengthUnits=m  SphereRadius=1  SphereRadiusUnits=m  EllipsoidRadii=[1 1 1]  EllipsoidRadiiUnits=m  ExtrusionCrossSection=[1 1; -1 1; -1 -1; 1 -1]  ExtrusionCrossSectionUnits=m  ExtrusionLength=1  ExtrusionLengthUnits=m  PolygonNumSides=3  PolygonOuterRadius=1  PolygonOuterRadiusUnits=m  ExtGeomFileType=STL  ExtGeomFileName=\STL\Right_Forearm.STL  ExtGeomFileUnits=mm  RevolutionCrossSection=[1 1; 1 -1; 2 -1; 2 1]  RevolutionCrossSectionUnits=m  RevolutionExtent=Full  RevolutionAngle=180  RevolutionAngleUnits=deg
  Right Elbow : PMIOPort  Side=Left
  EndEfector : PMIOPort  Port=2  Side=Right
  connections:
  Right Elbow/RConn1 -- Right Arm Endefector/LConn1 -- Solid/RConn1
  EndEfector/RConn1 -- Right Arm Endefector/RConn1

== system Robot/Robot simulation/Right Arm/Right Shoulder ==
  Right Shoulder Axis to Right Arm Base : sm_lib/Frames and Transforms/Rigid Transform  TranslationMethod=Cartesian  TranslationStandardOffset=0  TranslationLengthUnit=mm  TranslationStandardAxis=+Z  TranslationCartesianOffset=robot_right_shoulder_to_right_upper_arm_tra  TranslationROffset=0  TranslationROffsetUnits=m  TranslationZOffset=0  TranslationZOffsetUnits=m  TranslationThetaOffset=0  TranslationThetaOffsetUnits=deg  RotationMethod=RotationMatrix  RotationAngleUnits=deg  RotationStandardAxis=+Y  RotationAngle=270  RotationArbitraryAxis=[0 0 1]  FollAlignAxisA=+X  BaseAlignAxisA=+Y  FollAlignAxisB=+Y  BaseAlignAxisB=+Z  RotationSequenceAxes=FollowerAxes  RotationSequence=XYX  RotationSequenceAngles=[0 0 0]  RotationSequenceAnglesUnits=deg  RotationMatrix=robot_right_shoulder_to_right_upper_arm_rot
  Solid : sm_lib/Body Elements/Solid  InertiaType=Custom  Mass=robot_right_shoulder_mass  MassUnits=g  CenterOfMass=robot_right_shoulder_to_center_mass  CenterOfMassUnits=mm  MomentsOfInertia=robot_right_shoulder_moment_inertia  MomentsOfInertiaUnits=g*mm^2  ProductsOfInertia=robot_right_shoulder_product_inertia  ProductsOfInertiaUnits=g*mm^2  DensityBased=on  Density=1000  DensityUnits=kg/(m^3)  DoExposeReferenceFrame=on  SerializedFrames=<Frames/>  GraphicType=FromGeometry  MarkerShape=Sphere  MarkerSize=10  MarkerSizeUnits=m  GraphicVisPropType=SimpleVisualProperties  GraphicDiffuseColor=[0.5 0.5 0.5]  GraphicSpecularColor=[0.5 0.5 0.5 1.0]  GraphicAmbientColor=[0.15 0.15 0.15 1.0]  GraphicEmissiveColor=[0.0 0.0 0.0 1.0]  GraphicShininess=75  GraphicOpacity=1.0  GeometryShape=FromFile  RectangleSize=[1 1]  RectangleSizeUnits=m  BrickDimensions=[1 1 1]  BrickDimensionUnits=m  CylinderRadius=1  CylinderRadiusUnits=m  CylinderLength=1  CylinderLengthUnits=m  SphereRadius=1  SphereRadiusUnits=m  EllipsoidRadii=[1 1 1]  EllipsoidRadiiUnits=m  ExtrusionCrossSection=[1 1; -1 1; -1 -1; 1 -1]  ExtrusionCrossSectionUnits=m  ExtrusionLength=1  ExtrusionLengthUnits=m  PolygonNumSides=3  PolygonOuterRadius=1  PolygonOuterRadiusUnits=m  ExtGeomFileType=STL  ExtGeomFileName=\STL\Right_shoulder.STL  ExtGeomFileUnits=mm  RevolutionCrossSection=[1 1; 1 -1; 2 -1; 2 1]  RevolutionCrossSectionUnits=m  RevolutionExtent=Full  RevolutionAngle=180  RevolutionAngleUnits=deg
  Right Shoulder Pitch : PMIOPort  Side=Left
  Right Shoulder Roll : PMIOPort  Port=2  Side=Right
  connections:
  Solid/RConn1 -- Right Shoulder Pitch/RConn1 -- Right Shoulder Axis to Right Arm Base/LConn1
  Right Shoulder Axis to Right Arm Base/RConn1 -- Right Shoulder Roll/RConn1

== system Robot/Robot simulation/Right Arm/Right Shoulder Pitch (1) ==
  Inertia : sm_lib/Body Elements/Inertia  InertiaType=Custom  Mass=1  MassUnits=g  CenterOfMass=[0 0 0]  CenterOfMassUnits=m  MomentsOfInertia=[0 0 MX28_inertia]  MomentsOfInertiaUnits=kg*m^2  ProductsOfInertia=[0 0 0]  ProductsOfInertiaUnits=kg*m^2  GraphicType=Marker  MarkerShape=Inertia  MarkerSize=20  GraphicVisPropType=SimpleVisualProperties  GraphicDiffuseColor=[0.5 0.5 0.5]  GraphicSpecularColor=[0.5 0.5 0.5 1.0]  GraphicAmbientColor=[0.15 0.15 0.15 1.0]  GraphicEmissiveColor=[0.0 0.0 0.0 1.0]  GraphicShininess=75  GraphicOpacity=1.0
  MX28 Command : DataStoreRead  DataStoreName=MX28_ID1  SampleTime=MX28_Te  DataStoreElements=MX28_ID1.CW_angle_limit#MX28_ID1.CCW_angle_limit#MX28_ID1.torque_enable#MX28_ID1.D_gain#MX28_ID1.I_gain#MX28_ID1.P_gain#MX28_ID1.goal_position#MX28_ID1.moving_speed#MX28_ID1.torque_limit
  MX28 State : DataStoreWrite  DataStoreName=MX28_ID1  DataStoreElements=MX28_ID1.present_position#MX28_ID1.present_speed#MX28_ID1.present_load#MX28_ID1.moving#MX28_ID1.pwm
  Model : ModelReference  ModelNameDialog=MX28.slx  SimulationMode=Normal  ModelReferenceVersion=1.66
  Position converter : nesl_utility/PS-Simulink Converter  PhysicalDomain=network_engine_domain  SubClassName=ps_output  LeftPortType=input  RightPortType=output  PseudoPeriodic=off  Frequencies=[]  Unit=rad  AffineConversion=off
  Revolute Joint : sm_lib/Joints/Revolute Joint  SenseConstraintForce=off  SenseConstraintForceX=off  SenseConstraintForceY=off  SenseConstraintForceZ=off  SenseConstraintTorque=off  SenseConstraintTorqueX=off  SenseConstraintTorqueY=off  SenseConstraintTorqueZ=off  SenseTotalForce=off  SenseTotalForceX=off  SenseTotalForceY=off  SenseTotalForceZ=off  SenseTotalTorque=off  SenseTotalTorqueX=off  SenseTotalTorqueY=off  SenseTotalTorqueZ=off  CompositeWrenchDir=FollowerOnBase  CompositeWrenchFrame=BaseFrame  EquilibriumPosition=0  EquilibriumPositionUnits=deg  SpringStiffness=0  SpringStiffnessUnits=N*m/deg  DampingCoefficient=MX28_lub_friction  DampingCoefficientUnits=N*m/(rad/s)  TorqueActuationMode=InputTorque  MotionActuationMode=ComputedMotion  SensePosition=on  SenseVelocity=on  SenseAcceleration=off  SenseTorqueForce=off  PositionTargetSpecify=on  PositionTargetPriority=High  PositionTargetValue=MX28_init_position  PositionTargetValueUnits=rad  VelocityTargetSpecify=on  VelocityTargetPriority=High  VelocityTargetValue=MX28_init_speed  VelocityTargetValueUnits=rad/s
  Speed converter : nesl_utility/PS-Simulink Converter  PhysicalDomain=network_engine_domain  SubClassName=ps_output  LeftPortType=input  RightPortType=output  PseudoPeriodic=off  Frequencies=[]  Unit=rad/s  AffineConversion=off
  Torque converter : nesl_utility/Simulink-PS Converter  PhysicalDomain=network_engine_domain  SubClassName=ps_input  LeftPortType=input  RightPortType=output  PseudoPeriodic=off  Frequencies=[]  NoiseDistribution=none  NoiseParameters=[]  Unit=N*m  AffineConversion=off  FilteringAndDerivatives=zero  SimscapeFilterOrder=1  InputFilterTimeConstant=0.001  UdotUserProvided=1
  Base : PMIOPort  Side=Left
  Axis : PMIOPort  Port=2  Side=Right
  wires:
  Model/4 -> MX28 State/3
  Model/2 -> MX28 State/1
  Model/5 -> MX28 State/4
  Model/3 -> MX28 State/2
  MX28 Command/3 -> Model/5
  MX28 Command/6 -> Model/8
  MX28 Command/4 -> Model/6
  MX28 Command/5 -> Model/7
  MX28 Command/7 -> Model/9
  MX28 Command/2 -> Model/4
  MX28 Command/1 -> Model/3
  Speed converter/1 -> Model/1
  Position converter/1 -> Model/2
  Model/1 -> Torque converter/1
  Model/6 -> MX28 State/5
  MX28 Command/8 -> Model/10
  MX28 Command/9 -> Model/11
  connections:
  Axis/RConn1 -- Revolute Joint/RConn1 -- Inertia/RConn1
  Revolute Joint/LConn1 -- Base/RConn1
  Revolute Joint/RConn3 -- Speed converter/LConn1
  Revolute Joint/RConn2 -- Position converter/LConn1
  Revolute Joint/LConn2 -- Torque converter/RConn1
